simulink model "OCV_and_SOC_Estimation"  (R2024a)
settings: Solver=VariableStepAuto  StartTime=0.0  StopTime=10.0  RelTol=1e-3
settings Model: Creator=ACER  LastModifiedBy=ACER

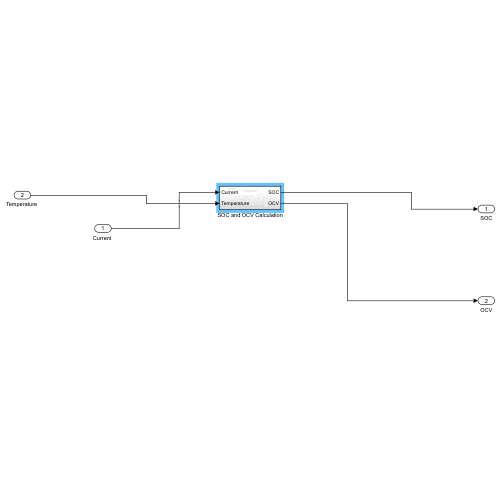
[thumbnail: Simulink's stored preview of the top-level diagram]
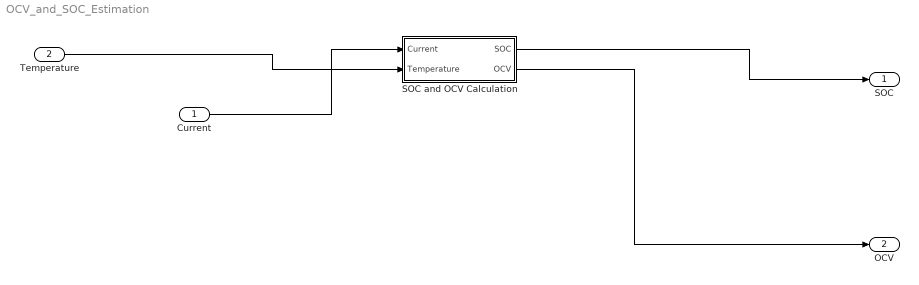
== system OCV_and_SOC_Estimation ==
  "Current " : Inport
  "Temperature " : Inport  Port=2
  SOC and OCV Calculation : Subsystem
  SOC : Outport
  OCV : Outport  Port=2
  wires:
  "Current "/1 -> SOC and OCV Calculation/1("Current ")
  "Temperature "/1 -> SOC and OCV Calculation/2("Temperature ")
  SOC and OCV Calculation/1(SOC) -> SOC/1
  SOC and OCV Calculation/2(OCV) -> OCV/1

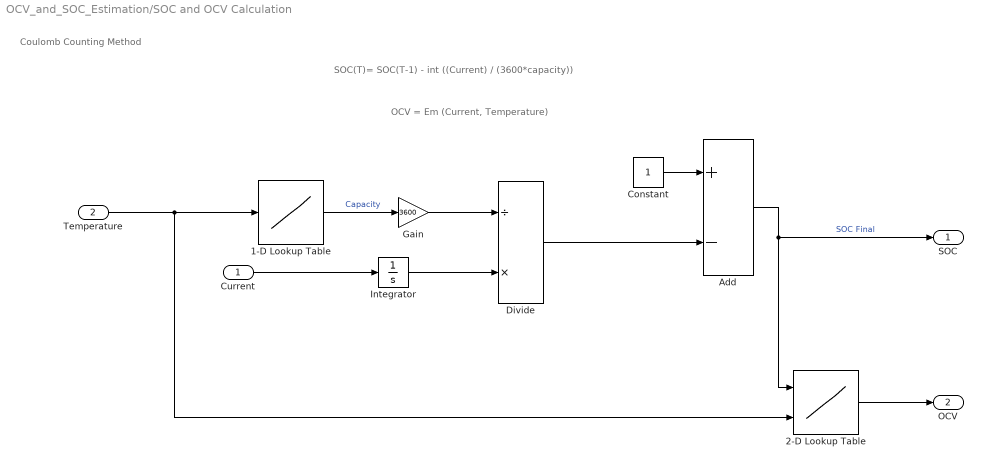
== system OCV_and_SOC_Estimation/SOC and OCV Calculation ==
  note: Coulomb Counting Method
  note: OCV = Em (Current, Temperature)
  note: SOC(T)= SOC(T-1) - int ((Current) / (3600*capacity))
  "Current " : Inport
  "Temperature " : Inport  Port=2
  1-D Lookup Table : Lookup_n-D  NumberOfTableDimensions=1  BreakpointsForDimension1=[-5:5]  Table=tanh([-5:5])  InternalRulePriority=Speed  RndMeth=Simplest
  2-D Lookup Table : Lookup_n-D  BreakpointsForDimension1=[1:3]  BreakpointsForDimension2=[1:3]  InternalRulePriority=Speed  RndMeth=Simplest
      settings: InputPortMap=u0,u1
  Add : Sum  Inputs=+-
  Constant : Constant
  Divide : Product  Inputs=/*
  Gain : Gain  Gain=3600
  Integrator : Integrator
  SOC : Outport
  OCV : Outport  Port=2
  wires:
  Integrator/1 -> Divide/2
  "Current "/1 -> Integrator/1
  1-D Lookup Table/1 -> Gain/1  "Capacity"
  Add/1 -> SOC/1, 2-D Lookup Table/1  "SOC Final"
  Gain/1 -> Divide/1
  Divide/1 -> Add/2
  "Temperature "/1 -> 2-D Lookup Table/2, 1-D Lookup Table/1
  Constant/1 -> Add/1
  2-D Lookup Table/1 -> OCV/1
